simulink model "bh_SL_test_car_and_CV_sys"  (R2017b)
settings: Solver=ode45  StartTime=0.0  StopTime=300  RelTol=1e-3
undefined symbols (not defined in the file or in its folder): gray, veh
libraries: simulink_extras x12, visiontextngfix x4, bh_cv_car_drc_library x2, visiongeotforms x1
settings Model: FPTRunName=Active  ExtModeAutoUpdateStatusClock=off  Creator=The MathWorks, Inc.  LastModifiedBy=bhorton
settings DataIOCC: LimitDataPoints=on  SaveFormat=Array  SaveOutput=off  SaveTime=off  SignalLoggingName=sigsOut
settings OptimizationCC: ExpressionDepthLimit=2147483647  InitFltsAndDblsToZero=on  LifeSpan=inf  BufferReusableBoundary=off
settings DebuggingCC: SaveWithParameterizedLinksMsg=none  UnderspecifiedInitializationDetection=Classic  MergeDetectMultiDrivingBlocksExec=none  CheckExecutionContextPreStartOutputMsg=on  CheckExecutionContextRuntimeOutputMsg=on  SignalResolutionControl=TryResolveAllWithWarning  MultiTaskDSMMsg=warning  MultiTaskCondExecSysMsg=none  ParameterPrecisionLossMsg=none  FcnCallInpInsideContextMsg=warning  BusObjectLabelMismatch=none  StateNameClashWarn=warning  StrictBusMsg=None  SFUnexpectedBacktrackingDiag=warning  SFNoUnconditionalDefaultTransitionDiag=warning  SFExecutionAtInitializationDiag=none
settings HardwareCC: ProdBitPerPointer=32  ProdBitPerSizeT=32  ProdBitPerPtrDiffT=32  ProdLargestAtomicFloat=None  ProdIntDivRoundTo=Undefined  ProdEndianess=Unspecified  ProdWordSize=32  ProdHWDeviceType=32-bit Generic  TargetBitPerPointer=64  TargetBitPerSizeT=64  TargetBitPerPtrDiffT=64  TargetLongLongMode=on  TargetIntDivRoundTo=Zero  TargetEndianess=LittleEndian  TargetWordSize=64  TargetHWDeviceType=Generic->MATLAB Host Computer  ProdEqTarget=off
settings ModelReferenceCC: PropagateSignalLabelsOutOfModel=off
settings CodeAppCC: StateflowObjectComments=on
settings GRTTargetCC: TargetFcnLib=ansi_tfl_tmw.mat  TargetLangStandard=C89/C90 (ANSI)  GeneratePreprocessorConditionals=Disable all  CombineOutputUpdateFcns=off  GRTInterface=on
settings ConfigComp: CovMetricSettings=dw  CovHtmlReporting=on  CovSaveCumulativeToWorkspaceVar=on  CovSaveSingleToWorkspaceVar=on  CovExternalEMLEnable=off

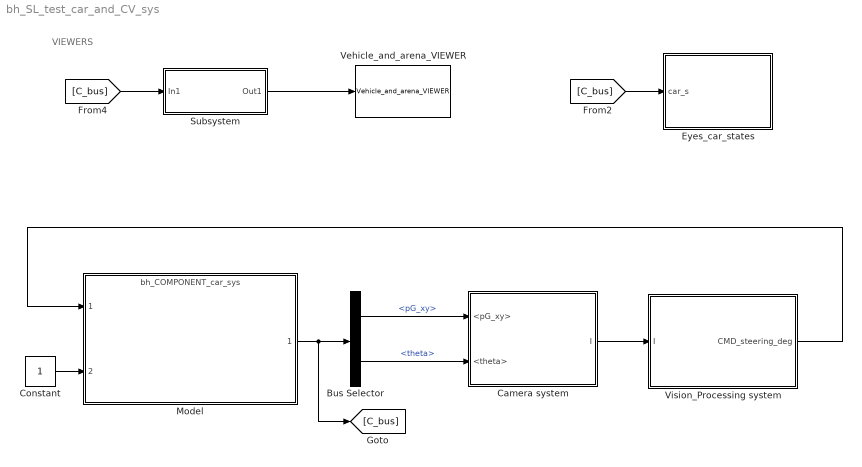
== system bh_SL_test_car_and_CV_sys ==
  note: VIEWERS
  Bus Selector : BusSelector  OutputSignals=states_G.pG_xy,states_B.theta
  Camera system : Subsystem
  Constant : Constant
  Eyes_car_states : Subsystem
  Model : ModelReference  ModelNameDialog=bh_COMPONENT_car_sys  SimulationMode=Normal  ModelReferenceVersion=1.271
  Subsystem : Subsystem
  Vehicle_and_arena_VIEWER : bh_cv_car_drc_library/CAR_things/Vehicle_and_arena_VIEWER  veh_ID_num=1  veh_init_xytheta=veh.states.init_pose  Ts=0.2
  Vision_Processing system : Subsystem
  wires:
  Model/1 -> [C_bus], Bus Selector/1
  Bus Selector/1 -> Camera system/1(<pG_xy>)  "<pG_xy>"
  Bus Selector/2 -> Camera system/2(<theta>)  "<theta>"
  Subsystem/1(Out1) -> Vehicle_and_arena_VIEWER/1
  [C_bus] -> Subsystem/1(In1)
  [C_bus] -> Eyes_car_states/1(car_s)
  Constant/1 -> Model/2
  Camera system/1(I) -> Vision_Processing system/1(I)
  Vision_Processing system/1(CMD_steering_deg) -> Model/1

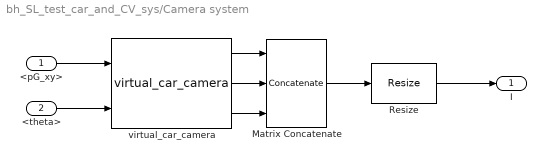
== system bh_SL_test_car_and_CV_sys/Camera system ==
  <pG_xy> : Inport
  <theta> : Inport  Port=2
  Matrix Concatenate : Concatenate  NumInputs=3  Mode=Multidimensional array  ConcatenateDimension=3
  Resize : visiongeotforms/Resize  specify=Number of output rows and columns  rfactor=[180 240]  outCols=25  outRows=25  outRowsCols=[240 320]  interp_method=Bilinear  antialias=off  useROI=off  roiFlag=off  prodOutputMode=Binary point scaling  prodOutputWordLength=32  prodOutputFracLength=10  roundingMode=Nearest  overflowMode=on
      settings: SourceProductName=Computer Vision System Toolbox  SourceProductBaseCode=VP
  virtual_car_camera : bh_cv_car_drc_library/CAR_things/virtual_car_camera  obstacle_visibility=SHOW_OBSTACLES  W=408  H=240  Ts=0.1  init_cam_pos_wrt_W=[veh.states.init_pos_G_Cxy(1), veh.states.init_pos_G_Cxy(2)]  height_of_cam=0.4  init_veh_THETA_wrt_W=0  horz_look_dist=111  cam_va=45
  I : Outport
  wires:
  Matrix Concatenate/1 -> Resize/1
  virtual_car_camera/3 -> Matrix Concatenate/3
  virtual_car_camera/1 -> Matrix Concatenate/1
  virtual_car_camera/2 -> Matrix Concatenate/2
  <theta>/1 -> virtual_car_camera/2
  <pG_xy>/1 -> virtual_car_camera/1
  Resize/1 -> I/1

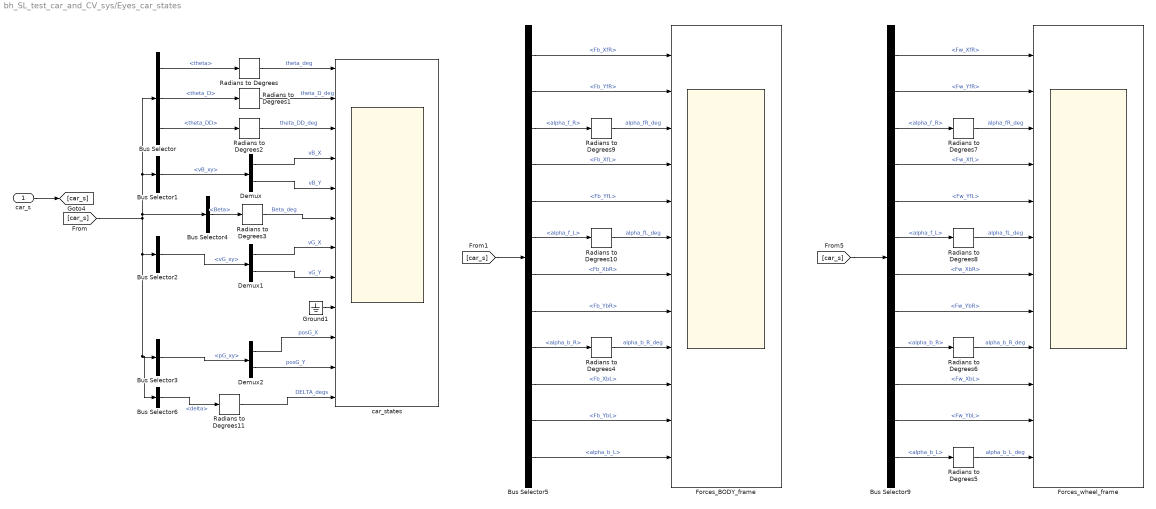
== system bh_SL_test_car_and_CV_sys/Eyes_car_states ==
  car_s : Inport
  Bus Selector : BusSelector  OutputSignals=states_B.theta,states_B.theta_D,states_B.theta_DD
  Bus Selector1 : BusSelector  OutputSignals=states_B.vB_xy
  Bus Selector2 : BusSelector  OutputSignals=states_G.vG_xy
  Bus Selector3 : BusSelector  OutputSignals=states_G.pG_xy
  Bus Selector4 : BusSelector  OutputSignals=states_B.Beta
  Bus Selector5 : BusSelector  OutputSignals=Force_BODY_frame.Fb_XfR,Force_BODY_frame.Fb_YfR,alpha.alpha_f_R,Force_BODY_frame.Fb_XfL,Force_BODY_frame.Fb_YfL,alpha.alpha_f_L,Force_BODY_frame.Fb_XbR,Force_BODY_frame.Fb_YbR,alpha.alpha_b_R,Force_BODY_frame.Fb_XbL,Force_BODY_frame.Fb_YbL,alpha.alpha_b_L
  Bus Selector6 : BusSelector  OutputSignals=wheel.delta
  Bus Selector9 : BusSelector  OutputSignals=Force_wheel_frame.Fw_XfR,Force_wheel_frame.Fw_YfR,alpha.alpha_f_R,Force_wheel_frame.Fw_XfL,Force_wheel_frame.Fw_YfL,alpha.alpha_f_L,Force_wheel_frame.Fw_XbR,Force_wheel_frame.Fw_YbR,alpha.alpha_b_R,Force_wheel_frame.Fw_XbL,Force_wheel_frame.Fw_YbL,alpha.alpha_b_L
  Demux : Demux  Outputs=2
  Demux1 : Demux  Outputs=2
  Demux2 : Demux  Outputs=2
  Forces_BODY_frame : Scope  NumInputPorts=12
  Forces_wheel_frame : Scope  NumInputPorts=12
  Ground1 : Ground
  Radians to Degrees{,1..11} (12 alike) : simulink_extras/Transformations/Radians to Degrees
  car_states : Scope  NumInputPorts=12
  wires:
  car_s/1 -> [car_s]
  [car_s] -> Bus Selector4/1, Bus Selector/1, Bus Selector1/1, Bus Selector6/1, Bus Selector3/1, Bus Selector2/1
  Bus Selector/1 -> Radians to Degrees/1  "<theta>"
  Bus Selector/2 -> Radians to Degrees1/1  "<theta_D>"
  Bus Selector/3 -> Radians to Degrees2/1  "<theta_DD>"
  Radians to Degrees/1 -> car_states/1  "theta_deg"
  Radians to Degrees1/1 -> car_states/2  "theta_D_deg"
  Radians to Degrees2/1 -> car_states/3  "theta_DD_deg"
  Bus Selector1/1 -> Demux/1  "<vB_xy>"
  Demux/1 -> car_states/4  "vB_X"
  Demux/2 -> car_states/5  "vB_Y"
  Radians to Degrees3/1 -> car_states/6  "Beta_deg"
  Bus Selector2/1 -> Demux1/1  "<vG_xy>"
  Demux1/1 -> car_states/7  "vG_X"
  Demux1/2 -> car_states/8  "vG_Y"
  Ground1/1 -> car_states/9
  Demux2/1 -> car_states/10  "posG_X"
  Demux2/2 -> car_states/11  "posG_Y"
  Bus Selector3/1 -> Demux2/1  "<pG_xy>"
  Radians to Degrees11/1 -> car_states/12  "DELTA_degs"
  Bus Selector4/1 -> Radians to Degrees3/1  "<Beta>"
  [car_s] -> Bus Selector9/1
  Bus Selector9/1 -> Forces_wheel_frame/1  "<Fw_XfR>"
  Bus Selector9/2 -> Forces_wheel_frame/2  "<Fw_YfR>"
  Bus Selector9/3 -> Radians to Degrees7/1  "<alpha_f_R>"
  Bus Selector9/4 -> Forces_wheel_frame/4  "<Fw_XfL>"
  Bus Selector9/5 -> Forces_wheel_frame/5  "<Fw_YfL>"
  Bus Selector9/6 -> Radians to Degrees8/1  "<alpha_f_L>"
  Bus Selector9/7 -> Forces_wheel_frame/7  "<Fw_XbR>"
  Bus Selector9/8 -> Forces_wheel_frame/8  "<Fw_YbR>"
  Bus Selector9/9 -> Radians to Degrees6/1  "<alpha_b_R>"
  Bus Selector9/10 -> Forces_wheel_frame/10  "<Fw_XbL>"
  Bus Selector9/11 -> Forces_wheel_frame/11  "<Fw_YbL>"
  Bus Selector9/12 -> Radians to Degrees5/1  "<alpha_b_L>"
  Radians to Degrees7/1 -> Forces_wheel_frame/3  "alpha_fR_deg"
  Radians to Degrees8/1 -> Forces_wheel_frame/6  "alpha_fL_deg"
  Radians to Degrees6/1 -> Forces_wheel_frame/9  "alpha_b_R_deg"
  Radians to Degrees5/1 -> Forces_wheel_frame/12  "alpha_b_L_deg"
  Radians to Degrees10/1 -> Forces_BODY_frame/6  "alpha_fL_deg"
  Radians to Degrees4/1 -> Forces_BODY_frame/9  "alpha_b_R_deg"
  Radians to Degrees9/1 -> Forces_BODY_frame/3  "alpha_fR_deg"
  Bus Selector5/9 -> Radians to Degrees4/1  "<alpha_b_R>"
  Bus Selector5/7 -> Forces_BODY_frame/7  "<Fb_XbR>"
  Bus Selector5/10 -> Forces_BODY_frame/10  "<Fb_XbL>"
  Bus Selector5/11 -> Forces_BODY_frame/11  "<Fb_YbL>"
  Bus Selector5/6 -> Radians to Degrees10/1  "<alpha_f_L>"
  Bus Selector5/5 -> Forces_BODY_frame/5  "<Fb_YfL>"
  Bus Selector5/4 -> Forces_BODY_frame/4  "<Fb_XfL>"
  Bus Selector5/8 -> Forces_BODY_frame/8  "<Fb_YbR>"
  Bus Selector5/2 -> Forces_BODY_frame/2  "<Fb_YfR>"
  [car_s] -> Bus Selector5/1
  Bus Selector5/3 -> Radians to Degrees9/1  "<alpha_f_R>"
  Bus Selector5/1 -> Forces_BODY_frame/1  "<Fb_XfR>"
  Bus Selector5/12 -> Forces_BODY_frame/12  "<alpha_b_L>"
  Bus Selector6/1 -> Radians to Degrees11/1  "<delta>"

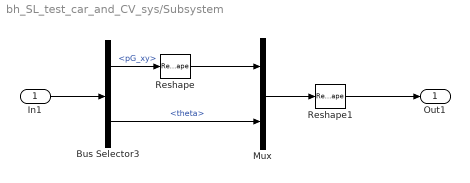
== system bh_SL_test_car_and_CV_sys/Subsystem ==
  In1 : Inport
  Bus Selector3 : BusSelector  OutputSignals=states_G.pG_xy,states_B.theta
  Mux : Mux  Inputs=2
  Reshape : Reshape  OutputDimensionality=Column vector (2-D)
  Reshape1 : Reshape  OutputDimensionality=Column vector (2-D)
  Out1 : Outport
  wires:
  In1/1 -> Bus Selector3/1
  Bus Selector3/1 -> Reshape/1  "<pG_xy>"
  Reshape/1 -> Mux/1
  Bus Selector3/2 -> Mux/2  "<theta>"
  Mux/1 -> Reshape1/1
  Reshape1/1 -> Out1/1

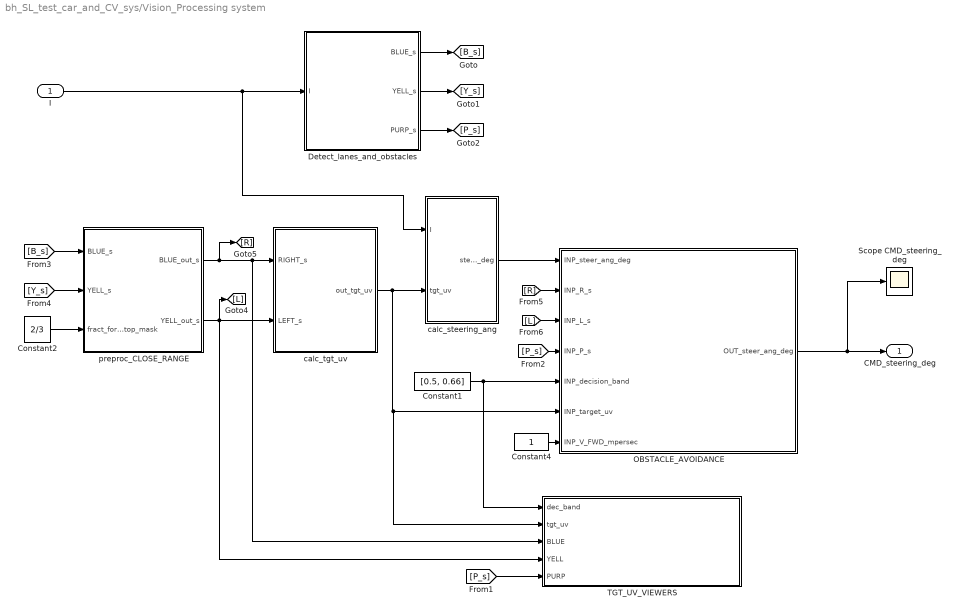
== system bh_SL_test_car_and_CV_sys/Vision_Processing system ==
  I : Inport
  Constant1 : Constant  Value=[0.5, 0.66]  OutDataTypeStr=double
  Constant2 : Constant  Value=2/3  OutDataTypeStr=double
  Constant4 : Constant  OutDataTypeStr=double
  Detect_lanes_and_obstacles : Subsystem
  OBSTACLE_AVOIDANCE : Stateflow chart  TreatAsAtomicUnit=on
  Scope CMD_steering_deg : Scope
  TGT_UV_VIEWERS : Subsystem
  calc_steering_ang : Subsystem
  calc_tgt_uv : MATLAB Function  TreatAsAtomicUnit=on
  preproc_CLOSE_RANGE : MATLAB Function  TreatAsAtomicUnit=on
  CMD_steering_deg : Outport
  wires:
  Detect_lanes_and_obstacles/2(YELL_s) -> [Y_s]
  [B_s] -> preproc_CLOSE_RANGE/1(BLUE_s)
  preproc_CLOSE_RANGE/1(BLUE_out_s) -> calc_tgt_uv/1(RIGHT_s), TGT_UV_VIEWERS/3(BLUE), [R]
  [P_s] -> TGT_UV_VIEWERS/5(PURP)
  Constant2/1 -> preproc_CLOSE_RANGE/3(fract_for_top_mask)
  Detect_lanes_and_obstacles/3(PURP_s) -> [P_s]
  Detect_lanes_and_obstacles/1(BLUE_s) -> [B_s]
  [Y_s] -> preproc_CLOSE_RANGE/2(YELL_s)
  preproc_CLOSE_RANGE/2(YELL_out_s) -> calc_tgt_uv/2(LEFT_s), [L], TGT_UV_VIEWERS/4(YELL)
  I/1 -> calc_steering_ang/1(I), Detect_lanes_and_obstacles/1(I)
  [P_s] -> OBSTACLE_AVOIDANCE/4(INP_P_s)
  [R] -> OBSTACLE_AVOIDANCE/2(INP_R_s)
  [L] -> OBSTACLE_AVOIDANCE/3(INP_L_s)
  calc_tgt_uv/1(out_tgt_uv) -> TGT_UV_VIEWERS/2(tgt_uv), OBSTACLE_AVOIDANCE/6(INP_target_uv), calc_steering_ang/2(tgt_uv)
  Constant4/1 -> OBSTACLE_AVOIDANCE/7(INP_V_FWD_mpersec)
  calc_steering_ang/1(steering_deg) -> OBSTACLE_AVOIDANCE/1(INP_steer_ang_deg)
  Constant1/1 -> TGT_UV_VIEWERS/1(dec_band), OBSTACLE_AVOIDANCE/5(INP_decision_band)
  OBSTACLE_AVOIDANCE/1(OUT_steer_ang_deg) -> Scope CMD_steering_deg/1, CMD_steering_deg/1

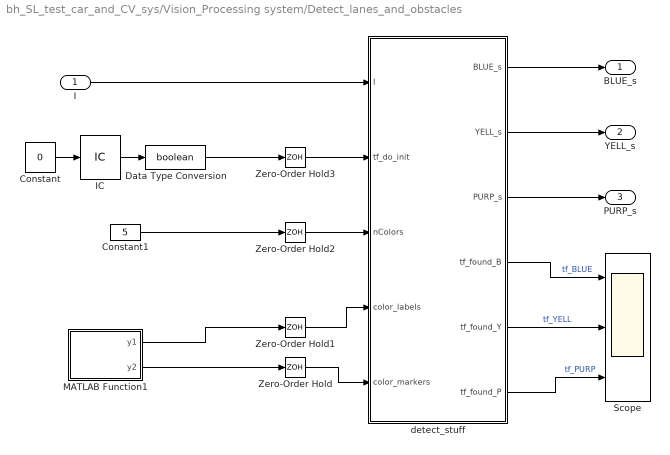
== system bh_SL_test_car_and_CV_sys/Vision_Processing system/Detect_lanes_and_obstacles ==
  I : Inport
  Constant : Constant  Value=0  OutDataTypeStr=boolean
  Constant1 : Constant  Value=5  OutDataTypeStr=double
  Data Type Conversion : DataTypeConversion  OutDataTypeStr=boolean
  IC : InitialCondition
  MATLAB Function1 : MATLAB Function  TreatAsAtomicUnit=on
  Scope : Scope  NumInputPorts=3
  Zero-Order Hold{,1..3} (4 alike) : ZeroOrderHold  SampleTime=0.1
  detect_stuff : MATLAB Function  TreatAsAtomicUnit=on
  BLUE_s : Outport
  YELL_s : Outport  Port=2
  PURP_s : Outport  Port=3
  wires:
  Constant/1 -> IC/1
  Data Type Conversion/1 -> Zero-Order Hold3/1
  IC/1 -> Data Type Conversion/1
  Constant1/1 -> Zero-Order Hold2/1
  MATLAB Function1/1(y1) -> Zero-Order Hold1/1
  MATLAB Function1/2(y2) -> Zero-Order Hold/1
  I/1 -> detect_stuff/1(I)
  detect_stuff/3(PURP_s) -> PURP_s/1
  detect_stuff/2(YELL_s) -> YELL_s/1
  detect_stuff/1(BLUE_s) -> BLUE_s/1
  Zero-Order Hold3/1 -> detect_stuff/2(tf_do_init)
  Zero-Order Hold2/1 -> detect_stuff/3(nColors)
  Zero-Order Hold1/1 -> detect_stuff/4(color_labels)
  Zero-Order Hold/1 -> detect_stuff/5(color_markers)
  detect_stuff/5(tf_found_Y) -> Scope/2  "tf_YELL"
  detect_stuff/4(tf_found_B) -> Scope/1  "tf_BLUE"
  detect_stuff/6(tf_found_P) -> Scope/3  "tf_PURP"

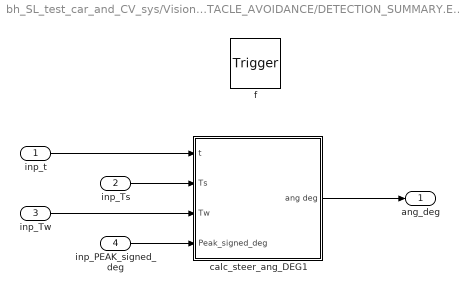
== system bh_SL_test_car_and_CV_sys/Vision_Processing system/OBSTACLE_AVOIDANCE/DETECTION_SUMMARY.EVASSIVE_MANOEUVRE.YES_DO_PERFORM.FUNC_calc_ang_deg ==
  inp_t : Inport  OutDataTypeStr=double  PortDimensions=1
  inp_Ts : Inport  Port=2  OutDataTypeStr=double  PortDimensions=1
  inp_Tw : Inport  Port=3  OutDataTypeStr=double  PortDimensions=1
  inp_PEAK_signed_deg : Inport  Port=4  OutDataTypeStr=double  PortDimensions=1
  f : TriggerPort  TriggerType=function-call  VariantControl=(inherit)
      settings: CopyFcn=Stateflow.SLINSF.SimulinkMan.removeBlockPreDeleteFcn  PreDeleteFcn=Stateflow.SLINSF.SimulinkMan.unsafePredeleteFcn
  calc_steer_ang_DEG1 : Subsystem
      mask Display: image(imread('evassive_PIC_01.JPG'))
  ang_deg : Outport
  wires:
  inp_t/1 -> calc_steer_ang_DEG1/1(t)
  calc_steer_ang_DEG1/1(ang deg) -> ang_deg/1
  inp_Tw/1 -> calc_steer_ang_DEG1/3(Tw)
  inp_PEAK_signed_deg/1 -> calc_steer_ang_DEG1/4(Peak_signed_deg)
  inp_Ts/1 -> calc_steer_ang_DEG1/2(Ts)

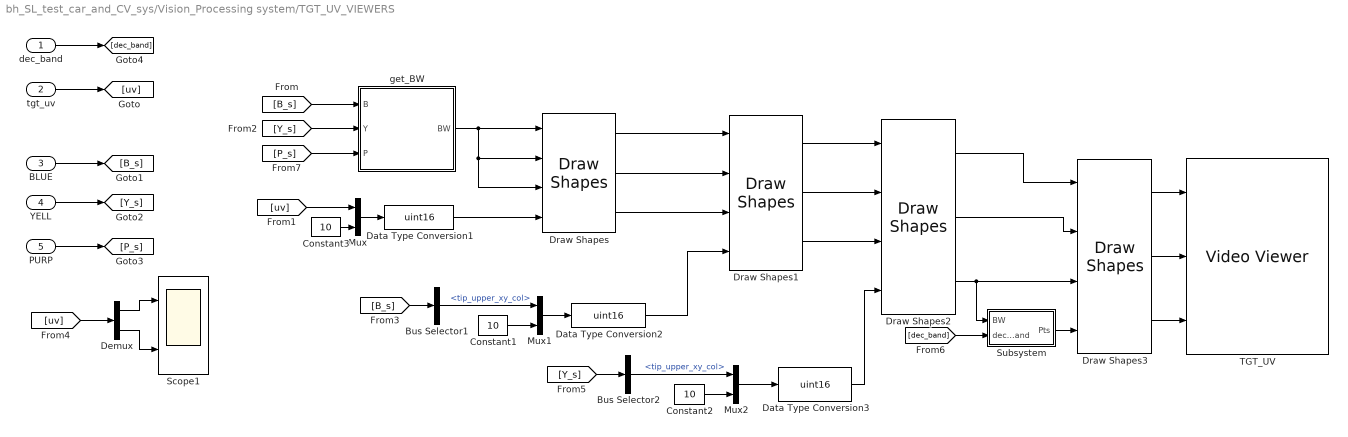
== system bh_SL_test_car_and_CV_sys/Vision_Processing system/TGT_UV_VIEWERS ==
  dec_band : Inport
  tgt_uv : Inport  Port=2
  BLUE : Inport  Port=3
  YELL : Inport  Port=4
  PURP : Inport  Port=5
  Bus Selector1 : BusSelector  OutputSignals=tip_upper_xy_col
  Bus Selector2 : BusSelector  OutputSignals=tip_upper_xy_col
  Constant1 : Constant  Value=10
  Constant2 : Constant  Value=10
  Constant3 : Constant  Value=10
  Data Type Conversion1 : DataTypeConversion  OutDataTypeStr=uint16
  Data Type Conversion2 : DataTypeConversion  OutDataTypeStr=uint16
  Data Type Conversion3 : DataTypeConversion  OutDataTypeStr=uint16
  Demux : Demux  Outputs=2
  Draw Shapes : visiontextngfix/Draw Shapes  shape=Circles  fill=on  lineWidth=1  fillClrSource=Specify via dialog  display=User-specified value  intensity=200  color=[255,0,0]  opacity=1  viewport=Entire image  antialiasing=off  inType=Obsolete  imagePorts=Separate color signals  prodOutputMode=Binary point scaling  prodOutputWordLength=32  prodOutputFracLength=14  memoryMode=Specify word length  memoryWordLength=16  memoryFracLength=14  roundingMode=Floor  overflowMode=off
      settings: SourceProductName=Computer Vision System Toolbox
  Draw Shapes1 : visiontextngfix/Draw Shapes  shape=Circles  fill=on  lineWidth=1  fillClrSource=Specify via dialog  display=User-specified value  intensity=200  color=[0,0,255]  opacity=1  viewport=Entire image  antialiasing=off  inType=Obsolete  imagePorts=Separate color signals  prodOutputMode=Binary point scaling  prodOutputWordLength=32  prodOutputFracLength=14  memoryMode=Specify word length  memoryWordLength=16  memoryFracLength=14  roundingMode=Floor  overflowMode=off
      settings: SourceProductName=Computer Vision System Toolbox
  Draw Shapes2 : visiontextngfix/Draw Shapes  shape=Circles  fill=on  lineWidth=1  fillClrSource=Specify via dialog  display=User-specified value  intensity=200  color=[255,255,0]  opacity=1  viewport=Entire image  antialiasing=off  inType=Obsolete  imagePorts=Separate color signals  prodOutputMode=Binary point scaling  prodOutputWordLength=32  prodOutputFracLength=14  memoryMode=Specify word length  memoryWordLength=16  memoryFracLength=14  roundingMode=Floor  overflowMode=off
      settings: SourceProductName=Computer Vision System Toolbox
  Draw Shapes3 : visiontextngfix/Draw Shapes  shape=Lines  fill=on  lineWidth=1  fillClrSource=Specify via dialog  display=User-specified value  intensity=200  color=[0,255,0]  opacity=1  viewport=Entire image  antialiasing=off  inType=Obsolete  imagePorts=Separate color signals  prodOutputMode=Binary point scaling  prodOutputWordLength=32  prodOutputFracLength=14  memoryMode=Specify word length  memoryWordLength=16  memoryFracLength=14  roundingMode=Floor  overflowMode=off
      settings: SourceProductName=Computer Vision System Toolbox
  Mux : Mux  Inputs=2
  Mux1 : Mux  Inputs=2
  Mux2 : Mux  Inputs=2
  Scope1 : Scope  NumInputPorts=2
  Subsystem : Subsystem
  TGT_UV : VideoViewer  imagePorts=separate color signals  colormapValue=gray(256)  FigPos=[1435 912 389 181]
  get_BW : Subsystem
  wires:
  Mux/1 -> Data Type Conversion1/1
  [uv] -> Mux/1
  Data Type Conversion1/1 -> Draw Shapes/4
  Constant3/1 -> Mux/2
  [P_s] -> get_BW/3(P)
  BLUE/1 -> [B_s]
  YELL/1 -> [Y_s]
  tgt_uv/1 -> [uv]
  [B_s] -> get_BW/1(B)
  [Y_s] -> get_BW/2(Y)
  PURP/1 -> [P_s]
  get_BW/1(BW) -> Draw Shapes/3, Draw Shapes/2, Draw Shapes/1
  Draw Shapes/1 -> Draw Shapes1/1
  Draw Shapes/2 -> Draw Shapes1/2
  Draw Shapes/3 -> Draw Shapes1/3
  [B_s] -> Bus Selector1/1
  Mux1/1 -> Data Type Conversion2/1
  Bus Selector1/1 -> Mux1/1  "<tip_upper_xy_col>"
  Constant1/1 -> Mux1/2
  Data Type Conversion2/1 -> Draw Shapes1/4
  Draw Shapes1/1 -> Draw Shapes2/1
  Draw Shapes1/2 -> Draw Shapes2/2
  Draw Shapes1/3 -> Draw Shapes2/3
  Constant2/1 -> Mux2/2
  Bus Selector2/1 -> Mux2/1  "<tip_upper_xy_col>"
  [Y_s] -> Bus Selector2/1
  Mux2/1 -> Data Type Conversion3/1
  Data Type Conversion3/1 -> Draw Shapes2/4
  [uv] -> Demux/1
  Demux/1 -> Scope1/1
  Demux/2 -> Scope1/2
  Draw Shapes3/1 -> TGT_UV/1
  Draw Shapes3/2 -> TGT_UV/2
  Draw Shapes3/3 -> TGT_UV/3
  Draw Shapes2/1 -> Draw Shapes3/1
  Draw Shapes2/2 -> Draw Shapes3/2
  Draw Shapes2/3 -> Subsystem/1(BW), Draw Shapes3/3
  dec_band/1 -> [dec_band]
  Subsystem/1(Pts) -> Draw Shapes3/4
  [dec_band] -> Subsystem/2(dec_band)

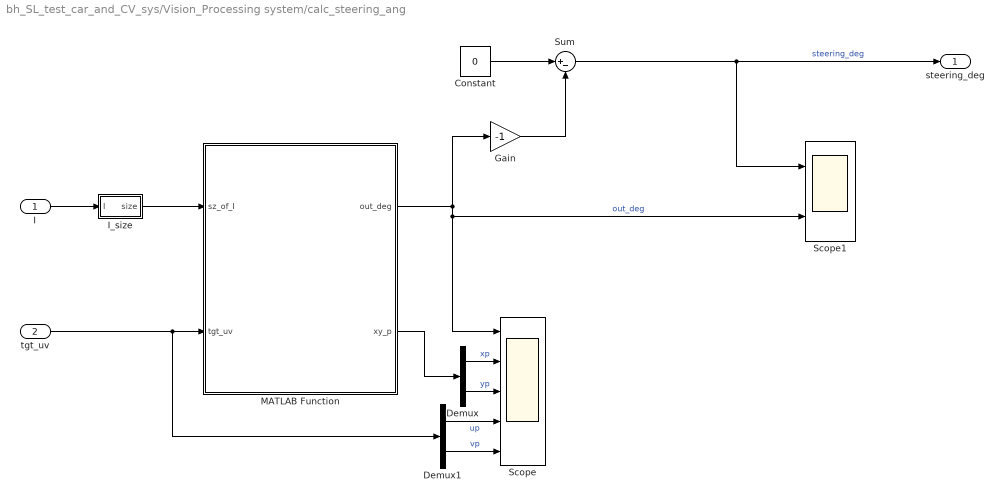
== system bh_SL_test_car_and_CV_sys/Vision_Processing system/calc_steering_ang ==
  I : Inport
  tgt_uv : Inport  Port=2
  Constant : Constant  Value=0
  Demux : Demux  Outputs=2
  Demux1 : Demux  Outputs=2
  Gain : Gain  Gain=-1
  I_size : Subsystem
  MATLAB Function : MATLAB Function  TreatAsAtomicUnit=on
  Scope : Scope  NumInputPorts=5
  Scope1 : Scope  NumInputPorts=2
  Sum : Sum  Inputs=|+-
  steering_deg : Outport
  wires:
  I/1 -> I_size/1(I)
  Sum/1 -> steering_deg/1, Scope1/1  "steering_deg"
  Demux1/1 -> Scope/4  "up"
  Constant/1 -> Sum/1
  Demux/2 -> Scope/3  "yp"
  Demux1/2 -> Scope/5  "vp"
  MATLAB Function/1(out_deg) -> Scope1/2, Scope/1, Gain/1  "out_deg"
  MATLAB Function/2(xy_p) -> Demux/1
  Gain/1 -> Sum/2
  Demux/1 -> Scope/2  "xp"
  tgt_uv/1 -> Demux1/1, MATLAB Function/2(tgt_uv)
  I_size/1(size) -> MATLAB Function/1(sz_of_I)

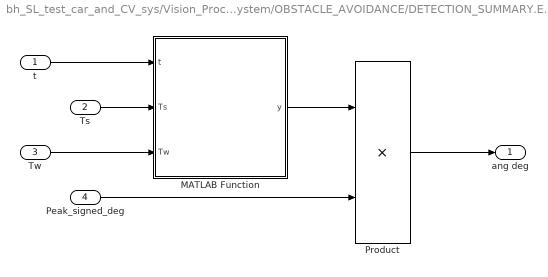
== system bh_SL_test_car_and_CV_sys/Vision_Processing system/OBSTACLE_AVOIDANCE/DETECTION_SUMMARY.EVASSIVE_MANOEUVRE.YES_DO_PERFORM.FUNC_calc_ang_deg/calc_steer_ang_DEG1 ==
  t : Inport
  Ts : Inport  Port=2
  Tw : Inport  Port=3
  Peak_signed_deg : Inport  Port=4
  MATLAB Function : MATLAB Function  TreatAsAtomicUnit=on
  Product : Product
  ang deg : Outport
  wires:
  t/1 -> MATLAB Function/1(t)
  Ts/1 -> MATLAB Function/2(Ts)
  Tw/1 -> MATLAB Function/3(Tw)
  MATLAB Function/1(y) -> Product/1
  Peak_signed_deg/1 -> Product/2
  Product/1 -> ang deg/1

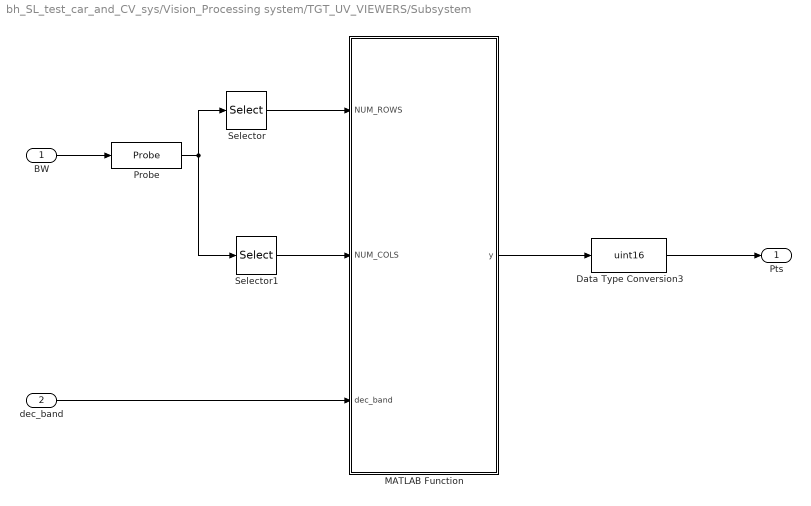
== system bh_SL_test_car_and_CV_sys/Vision_Processing system/TGT_UV_VIEWERS/Subsystem ==
  BW : Inport
  dec_band : Inport  Port=2
  Data Type Conversion3 : DataTypeConversion  OutDataTypeStr=uint16
  MATLAB Function : MATLAB Function  TreatAsAtomicUnit=on
  Probe : Probe  ProbeWidth=off  ProbeSampleTime=off  ProbeComplexSignal=off  ProbeSignalDimensions=on
  Selector : Selector  InputPortWidth=2  IndexOptions=Index vector (dialog)  Indices=1  OutputSizes=1
  Selector1 : Selector  InputPortWidth=2  IndexOptions=Index vector (dialog)  Indices=2  OutputSizes=1
  Pts : Outport
  wires:
  Probe/1 -> Selector1/1, Selector/1
  BW/1 -> Probe/1
  Selector/1 -> MATLAB Function/1(NUM_ROWS)
  Selector1/1 -> MATLAB Function/2(NUM_COLS)
  dec_band/1 -> MATLAB Function/3(dec_band)
  MATLAB Function/1(y) -> Data Type Conversion3/1
  Data Type Conversion3/1 -> Pts/1

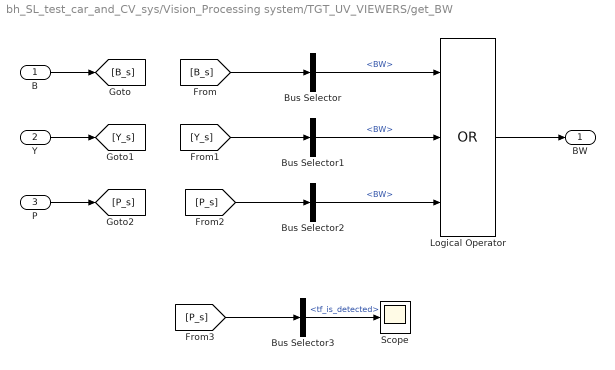
== system bh_SL_test_car_and_CV_sys/Vision_Processing system/TGT_UV_VIEWERS/get_BW ==
  B : Inport
  Y : Inport  Port=2
  P : Inport  Port=3
  Bus Selector : BusSelector  OutputSignals=BW
  Bus Selector1 : BusSelector  OutputSignals=BW
  Bus Selector2 : BusSelector  OutputSignals=BW
  Bus Selector3 : BusSelector  OutputSignals=tf_is_detected
  Logical Operator : Logic  Operator=OR  Inputs=3  AllPortsSameDT=off  OutDataTypeStr=boolean
  Scope : Scope
  BW : Outport
  wires:
  [P_s] -> Bus Selector2/1
  [B_s] -> Bus Selector/1
  Logical Operator/1 -> BW/1
  [Y_s] -> Bus Selector1/1
  Bus Selector/1 -> Logical Operator/1  "<BW>"
  Bus Selector1/1 -> Logical Operator/2  "<BW>"
  Bus Selector2/1 -> Logical Operator/3  "<BW>"
  P/1 -> [P_s]
  Y/1 -> [Y_s]
  B/1 -> [B_s]
  [P_s] -> Bus Selector3/1
  Bus Selector3/1 -> Scope/1  "<tf_is_detected>"

== system bh_SL_test_car_and_CV_sys/Vision_Processing system/calc_steering_ang/I_size ==
  I : Inport
  Probe : Probe  ProbeWidth=off  ProbeSampleTime=off  ProbeComplexSignal=off  ProbeSignalDimensions=on
  Selector : Selector  InputPortWidth=3  IndexOptions=Index vector (dialog)  Indices=[1 2]  OutputSizes=1
  size : Outport
  wires:
  Probe/1 -> Selector/1
  I/1 -> Probe/1
  Selector/1 -> size/1

== matlab function bh_SL_test_car_and_CV_sys/Vision_Processing system/OBSTACLE_AVOIDANCE/DETECTION_SUMMARY.EVASSIVE_MANOEUVRE.YES_DO_PERFORM.FUNC_calc_ang_deg/calc_steer_ang_DEG1/MATLAB Function ==
  data: t input; y output; Ts input; Tw input
function y = fcn(t,Ts,Tw)

y = 0;

% first look for the out of bounds cases
if(  t <= Ts )
    return;
end

if( t >= (Ts + 2*Tw) )
    return;
end

%OK: if we're here then do your thing
m_climbing = 1/(Tw/2);
m_falling  = -1 * m_climbing;

if(  (t > Ts) && (t <= (Ts + Tw/2))  )
    % first CLIMBING zone
    t_star = t - Ts;
         y = t_star * m_climbing;
elseif(  (t > (Ts + Tw/2)) && (t <= (Ts + 3*Tw/2))   )
    % the FALLING zone
    t_star = t - (Ts + Tw/2);
         y = t_star * m_falling +  1;
else
    % the 2nd CLIMBING zone
    t_star = t - (Ts + 3*Tw/2);
         y = t_star * m_climbing -  1;
end

== matlab function bh_SL_test_car_and_CV_sys/Vision_Processing system/TGT_UV_VIEWERS/Subsystem/MATLAB Function ==
  data: NUM_ROWS input; y output; NUM_COLS input; dec_band input
function y = fcn(NUM_ROWS, NUM_COLS, dec_band)

v_top = round( dec_band(1) * NUM_ROWS );
v_bot = round( dec_band(2) * NUM_ROWS );

y = [  1,  v_top, NUM_COLS, v_top;  
       1,  v_bot, NUM_COLS, v_bot; ];
   
end

== stateflow chart bh_SL_test_car_and_CV_sys/Vision_Processing system/OBSTACLE_AVOIDANCE ==
  state UTIL_FUNCS [group]
    note: ATTENTION:
        |
        | MATLAB functions within Stateflow charts can SEE local variables that are within SCOPE.
        | IFFF this is UNdesirable then do NOT define the MATLAB functions inside the StateFlow chart AND instead define them as
        | separate M-files.
  state tf_val_in_band = FUNC_is_OBST_in_band [function]
    note: Have we detected an obstacle ?
    note: ?
    note: are all of the obstacle pixels
        | underneath the BOTTOM decision
        | boundary OR are all of the obstacle pixes
        | above the TOP boundary
    (default) -> (junction 190)
    (junction 190) -> (junction 192) [order 1] : [false == INP_P_s.tf_is_detected]
    (junction 190) -> (junction 196) [order 2] : {
        |   % convert decision band into V co-ordinates
        |   v_top = round( INP_decision_band(1) * INP_P_s.NUM_ROWS );
        |   v_bot = round( INP_decision_band(2) * INP_P_s.NUM_ROWS );
        |
        |   v_bot_clear = round( 0.9 * INP_P_s.NUM_ROWS );
        |
        |   the_ind       = find(INP_P_s.BW);
        |   [tmp_y,tmp_x] = ind2sub(size( INP_P_s.BW),the_ind);
        |  }
    (junction 192) -> (junction 194) : {tf_val_in_band = false;}
    (junction 196) -> (junction 198)
    (junction 198) -> (junction 200) [order 1] : [  all(tmp_y > v_bot) ||  ...
        |    all(tmp_y < v_top)          ]
    (junction 198) -> (junction 205) [order 2] : {tf_val_in_band = true;}
    (junction 200) -> (junction 202) : { tf_val_in_band = false;}
    (junction 202) -> (junction 205)
    (junction 194) -> (junction 202)
    (junction 205) -> (junction 211)
  state DETECTION_SUMMARY
    state LEFT_LANE [parallel]
      settings: executionOrder=2
      state NOT_Detected
      state Detected
      (default) -> (junction 30)
      (junction 30) -> DETECTION_SUMMARY.LEFT_LANE.NOT_Detected [order 1] : [~INP_L_s.tf_is_detected]
      (junction 30) -> DETECTION_SUMMARY.LEFT_LANE.Detected [order 2] : [INP_L_s.tf_is_detected]
      DETECTION_SUMMARY.LEFT_LANE.NOT_Detected -> DETECTION_SUMMARY.LEFT_LANE.Detected : [INP_L_s.tf_is_detected]
      DETECTION_SUMMARY.LEFT_LANE.Detected -> DETECTION_SUMMARY.LEFT_LANE.NOT_Detected : [~INP_L_s.tf_is_detected]
    state RIGHT_LANE [parallel]
      settings: executionOrder=1
      state NOT_Detected
      state Detected
      (default) -> (junction 15)
      (junction 15) -> DETECTION_SUMMARY.RIGHT_LANE.NOT_Detected [order 1] : [~INP_R_s.tf_is_detected]
      (junction 15) -> DETECTION_SUMMARY.RIGHT_LANE.Detected [order 2] : [INP_R_s.tf_is_detected]
      DETECTION_SUMMARY.RIGHT_LANE.NOT_Detected -> DETECTION_SUMMARY.RIGHT_LANE.Detected : [INP_R_s.tf_is_detected]
      DETECTION_SUMMARY.RIGHT_LANE.Detected -> DETECTION_SUMMARY.RIGHT_LANE.NOT_Detected : [~INP_R_s.tf_is_detected]
    state OBSTACLE [parallel]
      settings: executionOrder=3
      state Detected
        state INSIDE_BAND
          en: tf_in_band = true;
        state OUTSIDE_BAND
          en: tf_in_band = false;
        (default) -> (junction 215)
        (junction 215) -> INSIDE_BAND [order 1] : [ FUNC_is_OBST_in_band() ]
        (junction 215) -> OUTSIDE_BAND [order 2]
        OUTSIDE_BAND -> INSIDE_BAND : [ FUNC_is_OBST_in_band() ]
        INSIDE_BAND -> OUTSIDE_BAND : [ ~FUNC_is_OBST_in_band()]
      state NOT_Detected
        en: tf_in_band = false;
      (default) -> (junction 41)
      (junction 41) -> DETECTION_SUMMARY.OBSTACLE.Detected [order 2] : [INP_P_s.tf_is_detected]
      (junction 41) -> DETECTION_SUMMARY.OBSTACLE.NOT_Detected [order 1] : [~INP_P_s.tf_is_detected]
      DETECTION_SUMMARY.OBSTACLE.NOT_Detected -> DETECTION_SUMMARY.OBSTACLE.Detected : [INP_P_s.tf_is_detected]
      DETECTION_SUMMARY.OBSTACLE.Detected -> DETECTION_SUMMARY.OBSTACLE.NOT_Detected : [~INP_P_s.tf_is_detected]
    state EVASSIVE_MANOEUVRE [parallel]
      settings: executionOrder=4
      state NO_DO_NOT_PERFORM
        entry, during:
        OUT_steer_ang_deg = INP_steer_ang_deg;
      state YES_DO_PERFORM
        entry:
        tf_have_finished_evasion = false;
        % determine profile of evassive manoeuvre
        Tstart = t;
        [tf_move_to_L, tf_move_to_R, gap_in_pix] = UTIL_FUNCS.quantify_evade(INP_target_uv, INP_decision_band, INP_P_s, INP_R_s, INP_L_s);
        y_offset_m = 0.3;
        PEAK_signed_deg = FUNC_calc_Peak_signed_deg();
        Tw = UTIL_FUNCS.calc_Tw(y_offset_m, INP_V_FWD_mpersec);
        entry, during:
        % calculate the steering angle of the evassive manoeuvre
        OUT_steer_ang_deg = FUNC_calc_ang_deg(t, Tstart, Tw, PEAK_signed_deg);
        FUNC_decide_if_finished();
        state ang_deg = FUNC_calc_ang_deg(inp_t,inp_Ts,inp_Tw,inp_PEAK_signed_deg) [function]
        state FUNC_decide_if_finished [function]
          (default) -> (junction 232)
          (junction 232) -> (junction 233) [order 1] : [t > (Tstart + 2*Tw)]
          (junction 232) -> (junction 234) [order 2]
          (junction 233) -> (junction 243) : { tf_have_finished_evasion = ...
              |   true; }
          (junction 234) -> (junction 235) : { tf_have_finished_evasion = ...
              |     false; }
          (junction 243) -> (junction 236)
          (junction 235) -> (junction 236)
          (junction 236) -> (junction 245)
        state y = FUNC_calc_Peak_signed_deg [function]
          (default) -> (junction 257)
          (junction 257) -> (junction 258) [order 1] : [tf_move_to_L]
          (junction 257) -> (junction 259) [order 2]
          (junction 258) -> (junction 265) : {k=1;}
          (junction 259) -> (junction 260) [order 1] : [tf_move_to_R]
          (junction 259) -> (junction 261) [order 2]
          (junction 260) -> (junction 264) : {k= - 1;}
          (junction 261) -> (junction 262)
          (junction 262) -> (junction 263) : {k = 0;}
          (junction 264) -> (junction 263)
          (junction 265) -> (junction 264)
          (junction 263) -> (junction 266) : {y = k * 25;}
      (default) -> NO_DO_NOT_PERFORM
      NO_DO_NOT_PERFORM -> (junction 223) : [ tf_in_band ]
      (junction 223) -> YES_DO_PERFORM : [ INP_L_s.tf_is_detected && ...
          |   INP_R_s.tf_is_detected ]
      (junction 225) -> NO_DO_NOT_PERFORM : [ ~tf_in_band ]
      YES_DO_PERFORM -> (junction 225) : [ (true==tf_have_finished_evasion)  ]
  (default) -> DETECTION_SUMMARY
  data: THE_Y_offset function_input; THE_Tw function_output; V_fwd_mpersec function_input; tf_move_to_left function_output; tf_move_to_right function_output; THE_gap_in_pix function_output; tgt_uv function_input; decision_band function_input; PURP_s function_input; RIGHT_s function_input; LEFT_s function_input; tf_val_in_band function_output; inp_t function_input double size=1; ang_deg function_output; inp_Ts function_input double size=1; inp_Tw function_input double size=1; inp_PEAK_signed_deg function_input double size=1; y function_output; gap_in_pix local; Tstart local; tf_move_to_L local boolean; tf_move_to_R local boolean; y_offset_m local; Tw local; PEAK_signed_deg local; tf_have_finished_evasion local; tf_in_band local boolean; INP_steer_ang_deg input double size=1; INP_R_s input Bus: lane_info_BUS; INP_L_s input Bus: lane_info_BUS; INP_P_s input Bus: box_info_BUS; INP_decision_band input double size=2; INP_target_uv input size=[2,1]; INP_V_FWD_mpersec input double size=1; OUT_steer_ang_deg output double size=1
  function THE_Tw = calc_Tw(THE_Y_offset, V_fwd_mpersec):
    | function THE_Tw = calc_Tw(THE_Y_offset, V_fwd_mpersec)
    | 
    | % make offset positive
    | THE_Y_offset = abs(THE_Y_offset);
    | 
    | % define lookup table data for V_forward = 1 m/sec
    | lookup_y  = 0.01 * [0,    4,  13,   30, 54];
    | lookup_Tw =        [0, 0.25, 0.5, 0.75,  1];
    | 
    | % scale y for the specified velocity
    | lookup_y = lookup_y * (V_fwd_mpersec/1)^2;
    | 
    | % ensure the supplied Y is in range
    | if(THE_Y_offset > max(lookup_y))
    |     THE_Y_offset = max(lookup_y);
    | end
    | 
    | % interpolate
    | THE_Tw = interp1(lookup_y, lookup_Tw, THE_Y_offset);
    | 
    | end
  function [tf_move_to_left, tf_move_to_right, THE_gap_in_pix] = quantify_evade(tgt_uv, decision_band, PURP_s, RIGHT_s, LEFT_s):
    | function [tf_move_to_left, tf_move_to_right, THE_gap_in_pix] = quantify_evade(tgt_uv, decision_band, PURP_s, RIGHT_s, LEFT_s) %#codegen
    | 
    | % default outputs
    | tf_move_to_left  = false;
    | tf_move_to_right = false;
    | THE_gap_in_pix   = 0;
    | 
    | 
    | % convert decision band into V co-ordinates
    | v_top = round( decision_band(1) * PURP_s.NUM_ROWS );
    | v_bot = round( decision_band(2) * PURP_s.NUM_ROWS );
    | 
    | 
    | % determine where our LEFT and RIGHT lanes intersect the decision bands
    | L_dband_s.tf_is_detected = LEFT_s.tf_is_detected;
    | L_dband_s.top_band_xy    = [0;v_top];
    | L_dband_s.bot_band_xy    = [0;v_bot];
    | L_dband_s.m              = LEFT_s.m;
    | L_dband_s.c              = LEFT_s.c;
    | 
    | R_dband_s.tf_is_detected = RIGHT_s.tf_is_detected;
    | R_dband_s.top_band_xy    = [0;v_top];
    | R_dband_s.bot_band_xy    = [0;v_bot];
    | R_dband_s.m              = RIGHT_s.m;
    | R_dband_s.c              = RIGHT_s.c;
    | 
    | if(L_dband_s.tf_is_detected)
    |     % V = m*U + c
    |     tmp_v = L_dband_s.top_band_xy(2);
    |     tmp_u = (tmp_v - LEFT_s.c)/LEFT_s.m;
    |     L_dband_s.top_band_xy(1) = tmp_u;
    |     
    |     tmp_v = L_dband_s.bot_band_xy(2);
    |     tmp_u = (tmp_v - LEFT_s.c)/LEFT_s.m;
    |     L_dband_s.bot_band_xy(1) = tmp_u;
    |     
    | end
    | 
    | if(R_dband_s.tf_is_detected)
    |     % V = m*U + c
    |     tmp_v = R_dband_s.top_band_xy(2);
    |     tmp_u = (tmp_v - RIGHT_s.c)/RIGHT_s.m;
    |     R_dband_s.top_band_xy(1) = tmp_u;
    |     
    |     tmp_v = R_dband_s.bot_band_xy(2);
    |     tmp_u = (tmp_v - RIGHT_s.c)/RIGHT_s.m;
    |     R_dband_s.bot_band_xy(1) = tmp_u;
    | end
    | 
    | % now make a decision
    | %++++++++++++++++++++++++++++++++++++++++++++++++++++++++++++++++++
    | if     (L_dband_s.tf_is_detected &&  R_dband_s.tf_is_detected)
    |     % BOTH detected
    |      [tf_move_to_left, tf_move_to_right, THE_gap_in_pix] = LOC_BOTH_detected(L_dband_s, R_dband_s, PURP_s, tgt_uv)    
    | elseif(L_dband_s.tf_is_detected )
    |     % only LEFT detected   #TODO
    |     
    | elseif(R_dband_s.tf_is_detected )
    |     % only RIGHT detected  #TODO
    | else
    |     % NONE detected
    |     return;
    | end
    | %++++++++++++++++++++++++++++++++++++++++++++++++++++++++++++++++++
    | 
    | 
    | end % calc_tgt_uv()
    | %==========================================================================
    | function [tf_move_to_left, tf_move_to_right, gap_in_pix] = LOC_BOTH_detected(L_dband_s, R_dband_s, PURP_s, INP_tgt_uv)
    | 
    |   % default outputs
    |   tf_move_to_left  = false;
    |   tf_move_to_right = false;
    |   gap_in_pix       = 0;
    |   
    |   % do your thing
    |   Uobst_L_edge  = PURP_s.left_edge_xy_col(1);
    |   Uobst_R_edge  = PURP_s.right_edge_xy_col(1);
    |   U_INP_tgt     = INP_tgt_uv(1);
    | 
    |   % do we have gaps between the lanes and the obstacle
    |   tf_left_side_gap  = false;  left_gap  = 0;
    |   tf_right_side_gap = false;  right_gap = 0;
    |   
    |   if(Uobst_L_edge > L_dband_s.bot_band_xy(1))
    |     tf_left_side_gap = true;
    |     left_gap = Uobst_L_edge - L_dband_s.bot_band_xy(1);
    |   end
    |   
    |   if(Uobst_R_edge < R_dband_s.bot_band_xy(1))
    |     tf_right_side_gap = true;
    |     right_gap = R_dband_s.bot_band_xy(1) - Uobst_R_edge;
    |   end
    |     
    |   % OK so we have a gap
    |   if(left_gap > right_gap)
    |       % left side gap is BIGGEST ... so move that way
    |       tf_move_to_left  = true;
    |       gap_in_pix       = left_gap;
    |   else
    |       % right side gap is BIGGEST ... so move that way
    |       tf_move_to_right  = true;
    |       gap_in_pix       = right_gap;
    |   end
    |       
    |       
    | end % LOC_BOTH_detected()
    | %_=========================================================================

== matlab function bh_SL_test_car_and_CV_sys/Vision_Processing system/Detect_lanes_and_obstacles/MATLAB Function1 ==
  data: y1 output; y2 output
function [y1, y2] = fcn()

y1 = [0,1,2,3,4];

y2 = [ ...
       -7.8436  -30.0394;
      -10.2908   36.4110;
       42.5297   -8.7231;
        2.1904    1.6907;
        4.0686    3.2113;
        ];
    
end

== matlab function bh_SL_test_car_and_CV_sys/Vision_Processing system/Detect_lanes_and_obstacles/detect_stuff ==
  data: I input; BLUE_s output Bus: lane_info_BUS; tf_do_init input; YELL_s output Bus: lane_info_BUS; PURP_s output Bus: box_info_BUS; nColors input; color_labels input; color_markers input; tf_found_B output boolean; tf_found_Y output boolean; tf_found_P output boolean
function [BLUE_s, YELL_s, PURP_s, tf_found_B, tf_found_Y, tf_found_P] = ...
         detect_stuff(I, tf_do_init, nColors, color_labels, color_markers)

coder.extrinsic('bh_my_detect_ALGORITHM_for_codegen')

marker_s.nColors       = nColors;
marker_s.color_labels  = color_labels;
marker_s.color_markers = color_markers;

[BLUE_s, YELL_s, PURP_s] = bh_my_detect_ALGORITHM_for_codegen(I, tf_do_init, marker_s);

tf_found_B = BLUE_s.tf_is_detected;
tf_found_Y = YELL_s.tf_is_detected;
tf_found_P = PURP_s.tf_is_detected;

end % detect_stuff()

== matlab function bh_SL_test_car_and_CV_sys/Vision_Processing system/calc_steering_ang/MATLAB Function ==
  data: sz_of_I input; tgt_uv input; out_deg output size=1; xy_p output
function [out_deg, xy_p]  = bh_calc_bearing_ang( sz_of_I, tgt_uv )


u_WIDTH  =  sz_of_I(2);
v_HEIGHT =  sz_of_I(1);

up = tgt_uv(1);
vp = tgt_uv(2);

out_rad = 0; 
out_deg = 0;

[ out_deg, xy_p ] = LOC_bh_calc_bearing_ang( up, vp, u_WIDTH, v_HEIGHT );

end
%_#########################################################################
function [out_deg, xy_p ] = LOC_bh_calc_bearing_ang( up, vp, u_WIDTH, v_HEIGHT )
% 
% Let:
%    W  = image width
%    H  = image height
%    up = u position of point P  relative to UV frame
%    vp = v position of point P  relative to UV frame
%
%     (0,0)                      A
%     0-------------------------|-------------------------->  U
%     |                         |
%     |                         ^  X
%     |                P  *     #
%     |                    \    #
%     |                     \   #
%     |                      \  #
%     |                       \ #
%     |                        \#      
%     |-------------<############-----------------------------
%  V  v              Y
%     
% Find:
%    the angle from the X axis to the point p (RH rule defines positive angle)
%--------------------------------------------------------------------------

H = v_HEIGHT;  W = u_WIDTH;

xp = H   - vp;
yp = W/2 - up;

out_rad = 0;
out_deg = 0;

out_rad = atan(yp/xp); 
out_deg = out_rad * 180/pi;

xy_p = [xp, yp];

% debug stuff
AA = 9;
if( ~isfinite(out_deg) )
    AA = 90;
else
    AA = 90;
end

end

== matlab function bh_SL_test_car_and_CV_sys/Vision_Processing system/calc_tgt_uv ==
  data: RIGHT_s input Bus: lane_info_BUS; LEFT_s input Bus: lane_info_BUS; out_tgt_uv output double
function out_tgt_uv = calc_tgt_uv(RIGHT_s,LEFT_s) %#codegen

out_tgt_uv = [0;0];

persistent tgt_uv
persistent C_to_L_dist
persistent C_to_R_dist

if( isempty(tgt_uv) )
    tgt_uv      = [LEFT_s.NUM_COLS/2; 1];
    C_to_L_dist = 0;
    C_to_R_dist = 0;
end

%++++++++++++++++++++++++++++++++++++++++++++++++++++++++++++++++++
if     (LEFT_s.tf_is_detected &&  RIGHT_s.tf_is_detected)
    % BOTH detected
    tgt_uv = LOC_BOTH_detected(LEFT_s, RIGHT_s);
    %%%tgt_uv = LOC_BOTH_detected_plan_B(LEFT_s, RIGHT_s);

    C_to_L_dist =  tgt_uv(1) -  LEFT_s.tip_upper_xy_col(1);
    C_to_R_dist =  tgt_uv(1) - RIGHT_s.tip_upper_xy_col(1);
    
elseif(LEFT_s.tf_is_detected &&  ~RIGHT_s.tf_is_detected)
    % only LEFT detected
    tgt_uv = LEFT_s.tip_upper_xy_col;
    tgt_uv(1) = tgt_uv(1) + abs(C_to_L_dist);
elseif(~LEFT_s.tf_is_detected &&   RIGHT_s.tf_is_detected)
    % only RIGHT detected
    tgt_uv = RIGHT_s.tip_upper_xy_col;
    tgt_uv(1) = tgt_uv(1) - abs(C_to_R_dist);
else
    % NONE detected
    tgt_uv = [LEFT_s.NUM_COLS/2; 1];
end
%++++++++++++++++++++++++++++++++++++++++++++++++++++++++++++++++++

if( ~all(isfinite(tgt_uv) )  )
    a  =78;
else
    a = 78;
end

%assert( all(isfinite(tgt_uv)), 'WHY NON finite in tgt_uv ??')


% take care of outputs
out_tgt_uv = tgt_uv;

end % calc_tgt_uv
%_#########################################################################
% END of MAIN function
%_#########################################################################
function tgt_uv = LOC_BOTH_detected(LEFT_s, RIGHT_s)

    % my_S.tip_upper_xy_col
    % my_S.tip_lower_xy_col
%     my_S.tip_upper_xy_col
%     my_S.tip_lower_xy_col

    tgt_uv    = [0;0];

    tgt_uv(1) = (LEFT_s.tip_upper_xy_col(1) + RIGHT_s.tip_upper_xy_col(1)) /2 ;
    tgt_uv(2) =  LEFT_s.tip_upper_xy_col(2);
end
%_=========================================================================
function tgt_uv = LOC_BOTH_detected_plan_B(LEFT_s, RIGHT_s)

    % my_S.tip_upper_xy_col
    % my_S.tip_lower_xy_col
%     my_S.tip_upper_xy_col
%     my_S.tip_lower_xy_col

    tgt_uv    = [0;0];

%     tgt_uv_A(1) = (LEFT_s.tip_upper_xy_col(1) + RIGHT_s.tip_upper_xy_col(1)) /2 ;
%     tgt_uv_A(2) =  LEFT_s.tip_upper_xy_col(2);
    
    v_lim = LOC_get_BOTH_vlimits(LEFT_s, RIGHT_s);
    u_lim = [1;LEFT_s.NUM_COLS];    
    
    if(any(v_lim <1) || any(u_lim<1) || any(~isfinite([v_lim;u_lim])))
        tmp=0;
    end
    
    % split vLIM into 3 equal bands
    NUM_BANDS = 3;
    v_bands   = round( linspace(v_lim(1), v_lim(2), (NUM_BANDS+1))  );
    
    tgt_uv_mat = zeros(2,NUM_BANDS);
    
    for kk=1:NUM_BANDS
        
        v_lim_local = [v_bands(kk); v_bands(kk+1)];
        u_lim_local = u_lim;
        v_range     = v_lim_local(1):v_lim_local(2); 
        
        BW_L =  zeros(  size(LEFT_s.BW )  ); 
        BW_R =  zeros(  size(RIGHT_s.BW)  );
        
        BW_L(v_range,:) = LEFT_s.BW(v_range,:);
        BW_R(v_range,:) = RIGHT_s.BW(v_range,:);
        
        L_O     = lane_info_CLS(BW_L, true);
        R_O     = lane_info_CLS(BW_R, true);

        L_O = L_O.calc_info(u_lim_local, v_lim_local);
        R_O = R_O.calc_info(u_lim_local, v_lim_local);
        
        L_s = L_O.convert_to_struct();
        R_s = R_O.convert_to_struct();
    
        tmp_tgt_uv = LOC_BOTH_detected(L_s, R_s);

        if( ~all(isfinite(tmp_tgt_uv)) )
            a = 90;
        else
            a = 78;
        end
        %assert( all(isfinite(tmp_tgt_uv)), 'WHY NON finite in TMP_tgt_uv ??')

        
        tgt_uv_mat(:,kk) = tmp_tgt_uv; 
    end
    
    % now do a weighted average
    tgt_uv = 10*tgt_uv_mat(:,1) + ...
             5*tgt_uv_mat(:,2) + ...
             2.5*tgt_uv_mat(:,3); 
    tgt_uv = tgt_uv/17.5;     
end
%_=========================================================================
function vlim = LOC_get_BOTH_vlimits(LEFT_s, RIGHT_s)

    % % get the lowest V top cordinate and bot co-ords
    % v_top = max( [LEFT_s.tip_upper_xy_col(2), RIGHT_s.tip_upper_xy_col(2)] );
    % v_bot = min( [LEFT_s.tip_lower_xy_col(2), RIGHT_s.tip_lower_xy_col(2)] );
    % 
    % vlim = [v_top; v_bot];

    the_ind   = find(LEFT_s.BW);
    [L_y,L_x] = ind2sub(size( LEFT_s.BW),the_ind); % convert INDS to SUBSCRIPTS

    the_ind   = find(RIGHT_s.BW);
    [R_y,R_x] = ind2sub(size(RIGHT_s.BW),the_ind); % convert INDS to SUBSCRIPTS

    v_top = max( [min(L_y), min(R_y)] );
    v_bot = min( [max(L_y), max(R_y)] );
    vlim = [v_top; v_bot];
end
%_=========================================================================
function tgt_uv = LOC_focus_on_RIGHT_only(RIGHT_s)
    tgt_uv    = [0;0];
    
    the_ind   = find(RIGHT_s.BW);
    [R_y,R_x] = ind2sub(size(RIGHT_s.BW),the_ind); % convert INDS to SUBSCRIPTS

    v_top = min(R_y);
    v_bot = max(R_y);
    v_lim = [v_top; v_bot];
    u_lim = [1;RIGHT_s.NUM_COLS];    
    
    if(any(v_lim <1) || any(u_lim<1) || any(~isfinite([v_lim;u_lim])))
        tmp=0;
    end
    
    % split vLIM into 3 equal bands
    NUM_BANDS = 3;
    v_bands   = round( linspace(v_lim(1), v_lim(2), (NUM_BANDS+1))  );
    
    tgt_uv_mat = zeros(2,NUM_BANDS);
    
    for kk=1:NUM_BANDS
        
        v_lim_local = [v_bands(kk); v_bands(kk+1)];
        u_lim_local = u_lim;
        v_range     = v_lim_local(1):v_lim_local(2); 
        
        BW_R =  zeros(  size(RIGHT_s.BW)  );        
        BW_R(v_range,:) = RIGHT_s.BW(v_range,:);
        
        R_O     = lane_info_CLS(BW_R, true);

        R_O = R_O.calc_info(u_lim_local, v_lim_local);
        R_s = R_O.convert_to_struct();
    
        tmp_tgt_uv = [0;0];
        tmp_tgt_uv(1) = RIGHT_s.tip_upper_xy_col(1);
        tmp_tgt_uv(2) = RIGHT_s.tip_upper_xy_col(2);
        
        if( ~all(isfinite(tmp_tgt_uv)) )
            a = 90;
        else
            a = 78;
        end
        %assert( all(isfinite(tmp_tgt_uv)), 'WHY NON finite in TMP_tgt_uv ??')
        
        tgt_uv_mat(:,kk) = tmp_tgt_uv; 
    end
    
    % now do a weighted average
    tgt_uv = 10*tgt_uv_mat(:,1) + ...
             5*tgt_uv_mat(:,2) + ...
             2.5*tgt_uv_mat(:,3); 
    tgt_uv = tgt_uv/17.5;     
end
%==========================================================================

== matlab function bh_SL_test_car_and_CV_sys/Vision_Processing system/preproc_CLOSE_RANGE ==
  data: BLUE_s input Bus: lane_info_BUS; YELL_s input Bus: lane_info_BUS; fract_for_top_mask input; BLUE_out_s output Bus: lane_info_BUS; YELL_out_s output Bus: lane_info_BUS
function [BLUE_out_s, YELL_out_s] = ...
     pre_process_lanes(BLUE_s, YELL_s, fract_for_top_mask) %#codegen

coder.extrinsic('bh_my_lane_preprocess_mask')

[BLUE_out_s, YELL_out_s] = ...
    bh_my_lane_preprocess_mask(BLUE_s, YELL_s, fract_for_top_mask);


end
